simulink model "Controller_ABS_VLC_AYC_ALGO2"  (Simulink 8.7)
settings: Solver=ode3  SolverMode=SingleTasking  StartTime=0.0  StopTime=6  FixedStep=0.001  RelTol=1e-3
undefined symbols (not defined in the file): Beta_Err_P_Gain, Cf, Cr, f_R_SA_cutoff, f_R_SA_cutoff_HP, f_WT_cutoff, f_YAW_cutoff, Fz, g, Kc1, Kc2, KX0, KX1, KX2, Lf, Lr, Lw, R_SA_Alpha_Gain, R_SA_Beta_Gain, R_SA_D_Gain, R_SA_P_Gain, SE_Alpha_Gain, SE_Beta_Gain, SE_D_Gain, SE_P_Gain, SR_Lim_n, SR_Lim_p, STA_BETA, STA_BETA_a, STA_DBETA, STA_DBETA_a, STA_DYE, STA_DYE_a, STA_OUT_K, STA_OUT_K_a, STA_OUT_K_BETA, STA_YE, STA_YE_a, T_Avail, Target_SR, Tau_Yaw, V_SA_D_Gain, V_SA_P_Gain, WT_P_Gain, YAW_Alpha_Gain, YAW_Beta_Gain, Yaw_Ctrl_Gain_SMCC, YAW_D_Gain, Yaw_Err_P_Gain, YAW_Int_Gain, YAW_P_Gain, YAW_Prop_Gain
libraries: dspindex x4
settings Model: MinMaxOverflowLogging=ForceOff  Creator=MR Spyder  LastModifiedBy=MR Spyder
settings DataIOCC: SignalLoggingSaveFormat=ModelDataLogs  SaveOutput=off  SaveTime=off
settings OptimizationCC: DefaultParameterBehavior=Inlined  ExpressionDepthLimit=2147483647
settings DebuggingCC: SolverPrmCheckMsg=warning  FcnCallInpInsideContextMsg=EnableAllAsWarning  StateNameClashWarn=warning
settings GRTTargetCC: CombineOutputUpdateFcns=off  GRTInterface=on

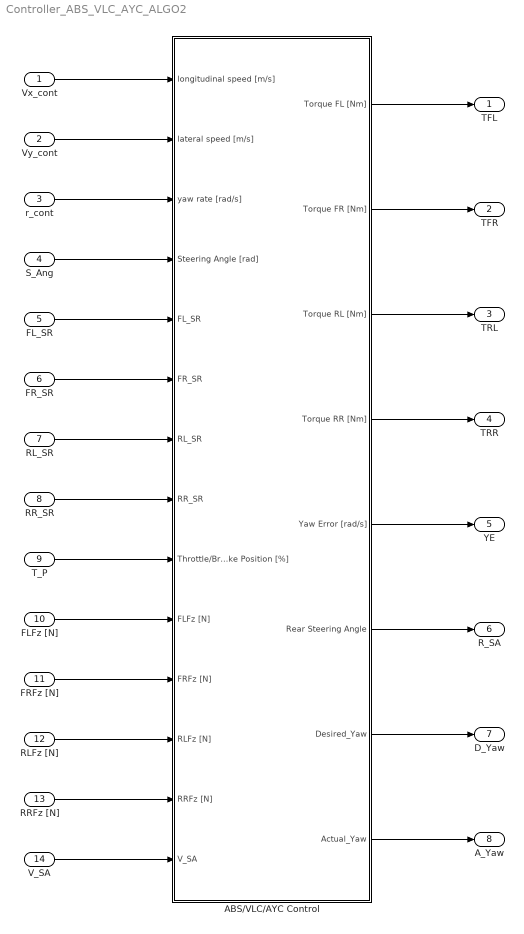
== system Controller_ABS_VLC_AYC_ALGO2 ==
  Vx_cont : Inport
  Vy_cont : Inport  Port=2
  r_cont : Inport  Port=3
  S_Ang : Inport  Port=4
  FL_SR : Inport  Port=5
  FR_SR : Inport  Port=6
  RL_SR : Inport  Port=7
  RR_SR : Inport  Port=8
  T_P : Inport  Port=9
  FLFz [N] : Inport  Port=10
  FRFz [N] : Inport  Port=11
  RLFz [N] : Inport  Port=12
  RRFz [N] : Inport  Port=13
  V_SA : Inport  Port=14
  ABS/VLC/AYC Control : Subsystem
  TFL : Outport
  TFR : Outport  Port=2
  TRL : Outport  Port=3
  TRR : Outport  Port=4
  YE : Outport  Port=5
  R_SA : Outport  Port=6
  D_Yaw : Outport  Port=7
  A_Yaw : Outport  Port=8
  wires:
  T_P/1 -> ABS/VLC/AYC Control/9(Throttle/Brake Position [%])
  ABS/VLC/AYC Control/1(Torque FL [Nm]) -> TFL/1
  ABS/VLC/AYC Control/2(Torque FR [Nm]) -> TFR/1
  ABS/VLC/AYC Control/3(Torque RL [Nm]) -> TRL/1
  ABS/VLC/AYC Control/4(Torque RR [Nm]) -> TRR/1
  FL_SR/1 -> ABS/VLC/AYC Control/5(FL_SR)
  FR_SR/1 -> ABS/VLC/AYC Control/6(FR_SR)
  RL_SR/1 -> ABS/VLC/AYC Control/7(RL_SR)
  RR_SR/1 -> ABS/VLC/AYC Control/8(RR_SR)
  r_cont/1 -> ABS/VLC/AYC Control/3(yaw rate [rad/s])
  Vy_cont/1 -> ABS/VLC/AYC Control/2(lateral speed [m/s])
  Vx_cont/1 -> ABS/VLC/AYC Control/1(longitudinal speed [m/s])
  S_Ang/1 -> ABS/VLC/AYC Control/4(Steering Angle [rad])
  ABS/VLC/AYC Control/5(Yaw Error [rad/s]) -> YE/1
  FLFz [N]/1 -> ABS/VLC/AYC Control/10(FLFz [N])
  FRFz [N]/1 -> ABS/VLC/AYC Control/11(FRFz [N])
  RLFz [N]/1 -> ABS/VLC/AYC Control/12(RLFz [N])
  RRFz [N]/1 -> ABS/VLC/AYC Control/13(RRFz [N])
  ABS/VLC/AYC Control/6(Rear Steering Angle) -> R_SA/1
  V_SA/1 -> ABS/VLC/AYC Control/14(V_SA)
  ABS/VLC/AYC Control/7(Desired_Yaw) -> D_Yaw/1
  ABS/VLC/AYC Control/8(Actual_Yaw) -> A_Yaw/1

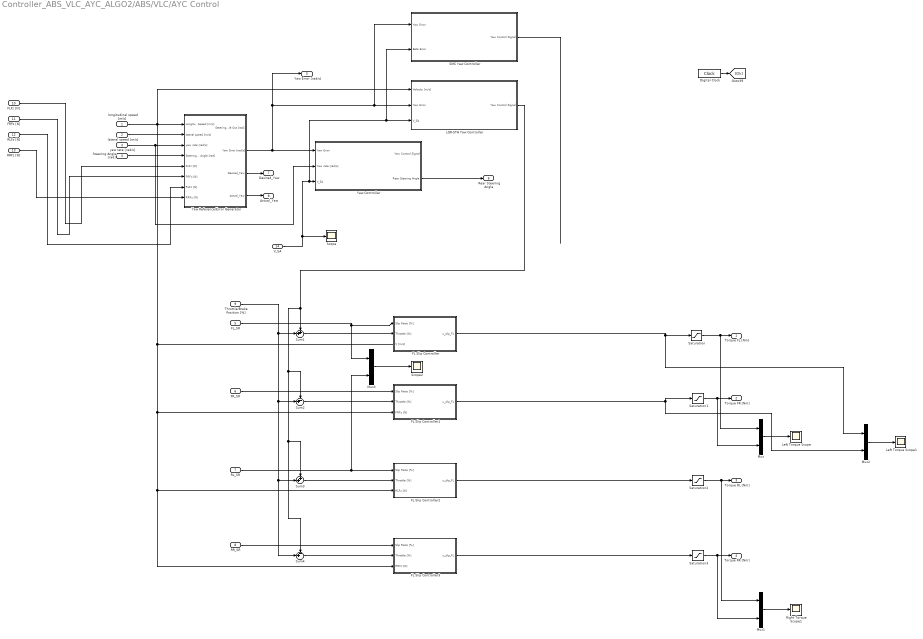
== system Controller_ABS_VLC_AYC_ALGO2/ABS/VLC/AYC Control ==
  longitudinal speed [m/s] : Inport
  lateral speed [m/s] : Inport  Port=2
  yaw rate [rad/s] : Inport  Port=3
  Steering Angle [rad] : Inport  Port=4
  FL_SR : Inport  Port=5
  FR_SR : Inport  Port=6
  RL_SR : Inport  Port=7
  RR_SR : Inport  Port=8
  Throttle/Brake Position [%] : Inport  Port=9
  FLFz [N] : Inport  Port=10
  FRFz [N] : Inport  Port=11
  RLFz [N] : Inport  Port=12
  RRFz [N] : Inport  Port=13
  V_SA : Inport  Port=14
  Digital Clock : DigitalClock  SampleTime=0.001
  FL Slip Controller : Subsystem
  FL Slip Controller1 : Subsystem
  FL Slip Controller2 : Subsystem
  FL Slip Controller3 : Subsystem
  LQR-STA Yaw Controller : Subsystem
  Left Torque Scope : Scope
  Left Torque Scope1 : Scope
  Mux{,1..3} (4 alike) : Mux  Inputs=2
  Right Torque Scope1 : Scope
  SMC Yaw Controller : Subsystem
  Saturation{,1..3} (4 alike) : Saturate  UpperLimit=T_Avail  LowerLimit=-T_Avail  LinearizeAsGain=off
  Scope : Scope
  Scope2 : Scope
  Sum1 : Sum  Inputs=++|
  Sum2 : Sum  Inputs=-+|
  Sum3 : Sum  Inputs=++|
  Sum4 : Sum  Inputs=-+|
  Yaw Controller : Subsystem
  Yaw Reference/Error Generator : Subsystem
  Torque FL [Nm] : Outport
  Torque FR [Nm] : Outport  Port=2
  Torque RL [Nm] : Outport  Port=3
  Torque RR [Nm] : Outport  Port=4
  Yaw Error [rad/s] : Outport  Port=5
  Rear Steering Angle : Outport  Port=6
  Desired_Yaw : Outport  Port=7
  Actual_Yaw : Outport  Port=8
  wires:
  Mux/1 -> Left Torque Scope/1
  Throttle/Brake Position [%]/1 -> Sum1/2, Sum2/2, Sum4/2, Sum3/2
  Mux1/1 -> Right Torque Scope1/1
  FL_SR/1 -> FL Slip Controller/1(Slip Ratio [%]), Mux3/1
  RL_SR/1 -> Mux3/2, FL Slip Controller2/1(Slip Ratio [%])
  RR_SR/1 -> FL Slip Controller3/1(Slip Ratio [%])
  Digital Clock/1 -> [Clk]
  FL Slip Controller/1(u_slip_FL) -> Mux2/1, Saturation/1
  FL Slip Controller1/1(u_slip_FL) -> Saturation1/1, Mux2/2
  FL Slip Controller2/1(u_slip_FL) -> Saturation2/1
  FL Slip Controller3/1(u_slip_FL) -> Saturation3/1
  LQR-STA Yaw Controller/1(Yaw Control Signal) -> Sum2/1, Sum3/1, Sum4/1, Sum1/1
  Saturation/1 -> Torque FL [Nm]/1, Mux/1
  Saturation1/1 -> Torque FR [Nm]/1, Mux/2
  Saturation2/1 -> Torque RL [Nm]/1, Mux1/1
  Saturation3/1 -> Torque RR [Nm]/1, Mux1/2
  Mux2/1 -> Left Torque Scope1/1
  Mux3/1 -> Scope2/1
  FR_SR/1 -> FL Slip Controller1/1(Slip Ratio [%])
  Sum1/1 -> FL Slip Controller/2(Throttle [%])
  Sum2/1 -> FL Slip Controller1/2(Throttle [%])
  Sum3/1 -> FL Slip Controller2/2(Throttle [%])
  Sum4/1 -> FL Slip Controller3/2(Throttle [%])
  yaw rate [rad/s]/1 -> Yaw Controller/2(Yaw rate [rad/s]), Yaw Reference/Error Generator/3(yaw rate [rad/s])
  Yaw Controller/2(Rear Steering Angle) -> Rear Steering Angle/1
  V_SA/1 -> Scope/1, SMC Yaw Controller/2(Beta Error), LQR-STA Yaw Controller/3(V_SA), Yaw Controller/3(V_SA)
  Yaw Reference/Error Generator/2(Yaw Error [rad/s]) -> Yaw Error [rad/s]/1, SMC Yaw Controller/1(Yaw Error), LQR-STA Yaw Controller/2(Yaw Error), Yaw Controller/1(Yaw Error)
  Yaw Reference/Error Generator/3(Desired_Yaw) -> Desired_Yaw/1
  Yaw Reference/Error Generator/4(Actual_Yaw) -> Actual_Yaw/1
  longitudinal speed [m/s]/1 -> FL Slip Controller1/3(FRFz [N]), FL Slip Controller3/3(RRFz [N]), FL Slip Controller2/3(RLFz [N]), LQR-STA Yaw Controller/1(Velocity [m/s]), Yaw Reference/Error Generator/1(Longitudinal Speed [m/s])
  lateral speed [m/s]/1 -> Yaw Reference/Error Generator/2(lateral speed [m/s])
  Steering Angle [rad]/1 -> Yaw Reference/Error Generator/4(Steering Angle [rad])
  FLFz [N]/1 -> Yaw Reference/Error Generator/5(FLFz [N])
  FRFz [N]/1 -> Yaw Reference/Error Generator/6(FRFz [N])
  RLFz [N]/1 -> Yaw Reference/Error Generator/7(RLFz [N])
  RRFz [N]/1 -> Yaw Reference/Error Generator/8(RRFz [N])
  SMC Yaw Controller/1(Yaw Control Signal) -> ?

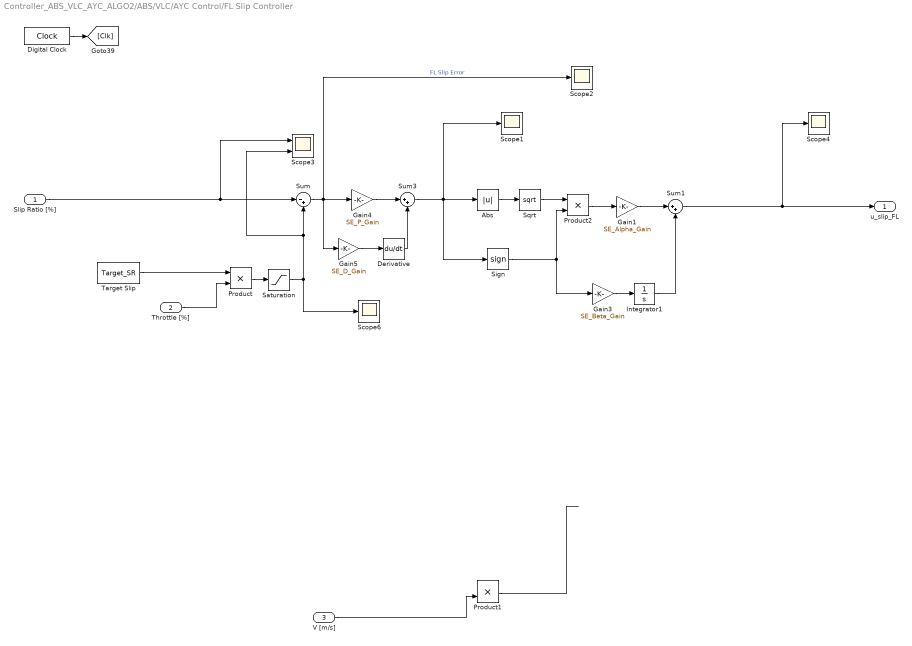
== system Controller_ABS_VLC_AYC_ALGO2/ABS/VLC/AYC Control/FL Slip Controller ==
  Slip Ratio [%] : Inport
  Throttle [%] : Inport  Port=2
  V [m/s] : Inport  Port=3
  Abs : Abs
  Derivative : Derivative
  Digital Clock : DigitalClock  SampleTime=0.001
  Gain1 : Gain  Gain=SE_Alpha_Gain
  Gain3 : Gain  Gain=SE_Beta_Gain
  Gain4 : Gain  Gain=SE_P_Gain
  Gain5 : Gain  Gain=SE_D_Gain
  Integrator1 : Integrator
  Product : Product
  Product1 : Product
  Product2 : Product
  Saturation : Saturate  UpperLimit=SR_Lim_p  LowerLimit=SR_Lim_n  LinearizeAsGain=off
  Scope{1..2,4,6} (4 alike) : Scope
  Scope3 : Scope  NumInputPorts=2
  Sign : Signum
  Sqrt : Sqrt  SaturateOnIntegerOverflow=on
  Sum : Sum  Inputs=|-+
  Sum1 : Sum  Inputs=|++
  Sum3 : Sum  Inputs=|++
  Target Slip : Constant  Value=Target_SR
  u_slip_FL : Outport
  wires:
  Digital Clock/1 -> [Clk]
  Sqrt/1 -> Product2/1
  Sum1/1 -> Scope4/1, u_slip_FL/1
  Slip Ratio [%]/1 -> Sum/1, Scope3/1
  Throttle [%]/1 -> Product/2
  Product/1 -> Saturation/1
  Target Slip/1 -> Product/1
  Sum/1 -> Gain5/1, Gain4/1, Scope2/1  "FL Slip Error"
  Product2/1 -> Gain1/1
  Abs/1 -> Sqrt/1
  Sign/1 -> Gain3/1, Product2/2
  Sum3/1 -> Scope1/1, Sign/1, Abs/1
  Integrator1/1 -> Sum1/2
  Gain1/1 -> Sum1/1
  Gain3/1 -> Integrator1/1
  Gain4/1 -> Sum3/1
  Derivative/1 -> Sum3/2
  Gain5/1 -> Derivative/1
  Saturation/1 -> Scope6/1, Scope3/2, Sum/2
  ? -> Product1/1
  V [m/s]/1 -> Product1/2
  Product1/1 -> ?

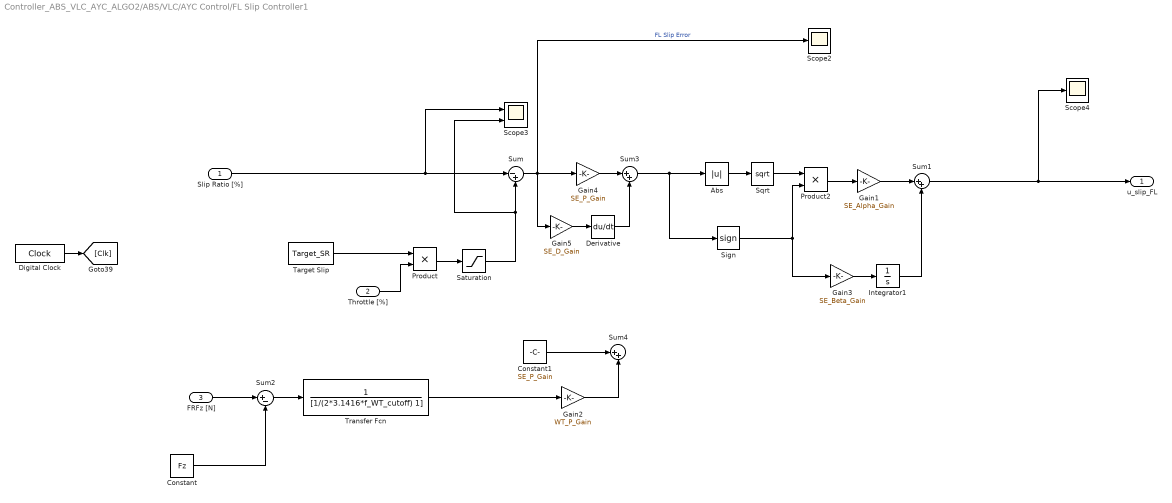
== system Controller_ABS_VLC_AYC_ALGO2/ABS/VLC/AYC Control/FL Slip Controller1 ==
  Slip Ratio [%] : Inport
  Throttle [%] : Inport  Port=2
  FRFz [N] : Inport  Port=3
  Abs : Abs
  Constant : Constant  Value=Fz
  Constant1 : Constant  Value=SE_P_Gain
  Derivative : Derivative
  Digital Clock : DigitalClock  SampleTime=0.001
  Gain1 : Gain  Gain=SE_Alpha_Gain
  Gain2 : Gain  Gain=WT_P_Gain
  Gain3 : Gain  Gain=SE_Beta_Gain
  Gain4 : Gain  Gain=SE_P_Gain
  Gain5 : Gain  Gain=SE_D_Gain
  Integrator1 : Integrator
  Product : Product
  Product2 : Product
  Saturation : Saturate  UpperLimit=SR_Lim_p  LowerLimit=SR_Lim_n  LinearizeAsGain=off
  Scope2 : Scope
  Scope3 : Scope  NumInputPorts=2
  Scope4 : Scope
  Sign : Signum
  Sqrt : Sqrt  SaturateOnIntegerOverflow=on
  Sum : Sum  Inputs=|-+
  Sum1 : Sum  Inputs=|++
  Sum2 : Sum  Inputs=|+-
  Sum3 : Sum  Inputs=|++
  Sum4 : Sum  Inputs=|++
  Target Slip : Constant  Value=Target_SR
  Transfer Fcn : TransferFcn  Denominator=[1/(2*3.1416*f_WT_cutoff) 1]
  u_slip_FL : Outport
  wires:
  Sqrt/1 -> Product2/1
  Digital Clock/1 -> [Clk]
  Sum1/1 -> Scope4/1, u_slip_FL/1
  Slip Ratio [%]/1 -> Sum/1, Scope3/1
  Throttle [%]/1 -> Product/2
  Product/1 -> Saturation/1
  Target Slip/1 -> Product/1
  FRFz [N]/1 -> Sum2/1
  Transfer Fcn/1 -> Gain2/1
  Constant/1 -> Sum2/2
  Sum2/1 -> Transfer Fcn/1
  Sum/1 -> Gain5/1, Gain4/1, Scope2/1  "FL Slip Error"
  Gain2/1 -> Sum4/2
  Constant1/1 -> Sum4/1
  Product2/1 -> Gain1/1
  Abs/1 -> Sqrt/1
  Sign/1 -> Product2/2, Gain3/1
  Derivative/1 -> Sum3/2
  Sum3/1 -> Sign/1, Abs/1
  Integrator1/1 -> Sum1/2
  Gain1/1 -> Sum1/1
  Gain3/1 -> Integrator1/1
  Gain4/1 -> Sum3/1
  Gain5/1 -> Derivative/1
  Saturation/1 -> Scope3/2, Sum/2

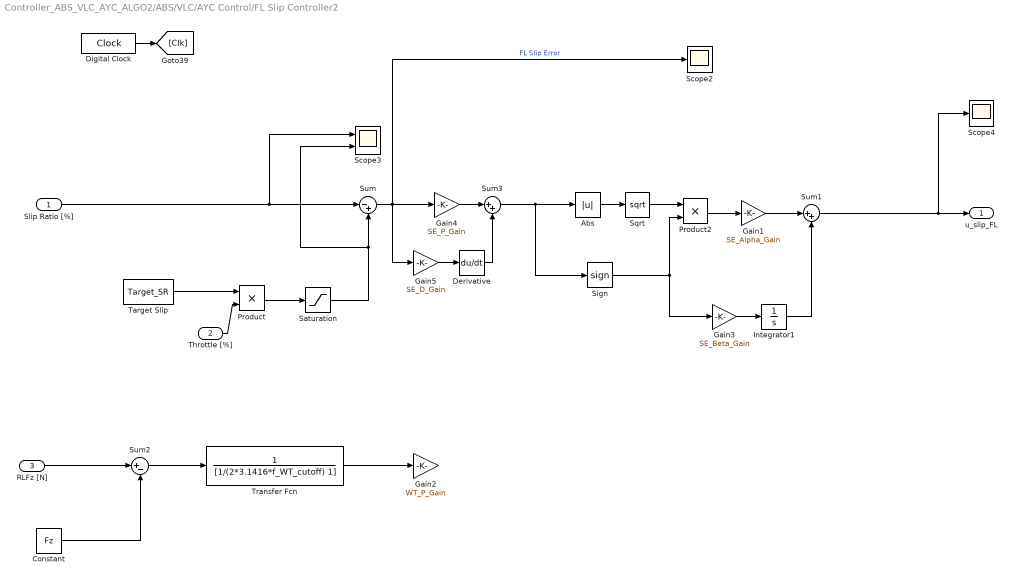
== system Controller_ABS_VLC_AYC_ALGO2/ABS/VLC/AYC Control/FL Slip Controller2 ==
  Slip Ratio [%] : Inport
  Throttle [%] : Inport  Port=2
  RLFz [N] : Inport  Port=3
  Abs : Abs
  Constant : Constant  Value=Fz
  Derivative : Derivative
  Digital Clock : DigitalClock  SampleTime=0.001
  Gain1 : Gain  Gain=SE_Alpha_Gain
  Gain2 : Gain  Gain=WT_P_Gain
  Gain3 : Gain  Gain=SE_Beta_Gain
  Gain4 : Gain  Gain=SE_P_Gain
  Gain5 : Gain  Gain=SE_D_Gain
  Integrator1 : Integrator
  Product : Product
  Product2 : Product
  Saturation : Saturate  UpperLimit=SR_Lim_p  LowerLimit=SR_Lim_n  LinearizeAsGain=off
  Scope2 : Scope
  Scope3 : Scope  NumInputPorts=2
  Scope4 : Scope
  Sign : Signum
  Sqrt : Sqrt  SaturateOnIntegerOverflow=on
  Sum : Sum  Inputs=|-+
  Sum1 : Sum  Inputs=|++
  Sum2 : Sum  Inputs=|+-
  Sum3 : Sum  Inputs=|++
  Target Slip : Constant  Value=Target_SR
  Transfer Fcn : TransferFcn  Denominator=[1/(2*3.1416*f_WT_cutoff) 1]
  u_slip_FL : Outport
  wires:
  Digital Clock/1 -> [Clk]
  RLFz [N]/1 -> Sum2/1
  Transfer Fcn/1 -> Gain2/1
  Constant/1 -> Sum2/2
  Sum2/1 -> Transfer Fcn/1
  Sqrt/1 -> Product2/1
  Sum1/1 -> u_slip_FL/1, Scope4/1
  Slip Ratio [%]/1 -> Sum/1, Scope3/1
  Throttle [%]/1 -> Product/2
  Product/1 -> Saturation/1
  Target Slip/1 -> Product/1
  Sum/1 -> Gain5/1, Gain4/1, Scope2/1  "FL Slip Error"
  Product2/1 -> Gain1/1
  Abs/1 -> Sqrt/1
  Sign/1 -> Product2/2, Gain3/1
  Derivative/1 -> Sum3/2
  Sum3/1 -> Sign/1, Abs/1
  Integrator1/1 -> Sum1/2
  Gain1/1 -> Sum1/1
  Gain3/1 -> Integrator1/1
  Gain4/1 -> Sum3/1
  Gain5/1 -> Derivative/1
  Saturation/1 -> Scope3/2, Sum/2

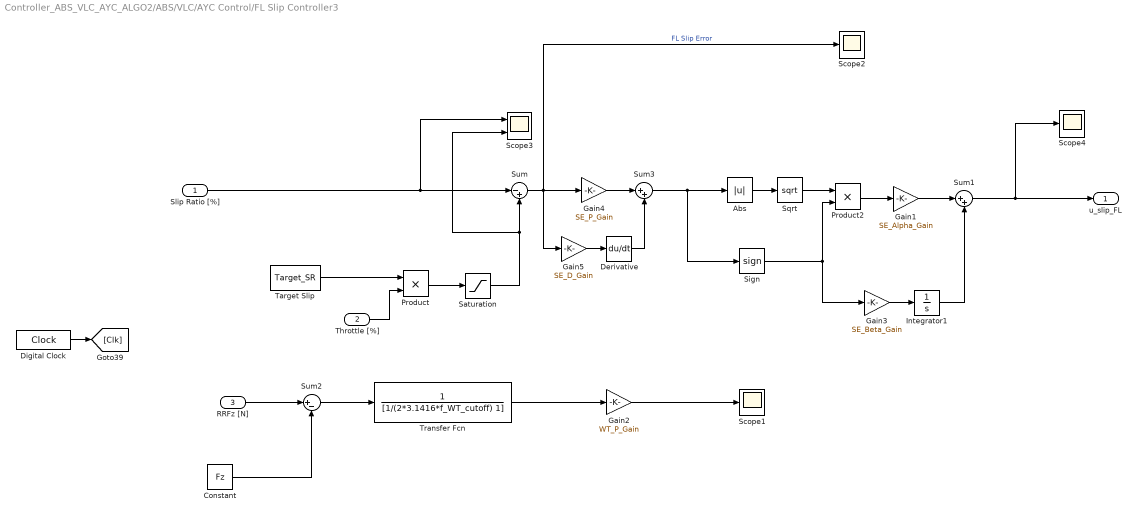
== system Controller_ABS_VLC_AYC_ALGO2/ABS/VLC/AYC Control/FL Slip Controller3 ==
  Slip Ratio [%] : Inport
  Throttle [%] : Inport  Port=2
  RRFz [N] : Inport  Port=3
  Abs : Abs
  Constant : Constant  Value=Fz
  Derivative : Derivative
  Digital Clock : DigitalClock  SampleTime=0.001
  Gain1 : Gain  Gain=SE_Alpha_Gain
  Gain2 : Gain  Gain=WT_P_Gain
  Gain3 : Gain  Gain=SE_Beta_Gain
  Gain4 : Gain  Gain=SE_P_Gain
  Gain5 : Gain  Gain=SE_D_Gain
  Integrator1 : Integrator
  Product : Product
  Product2 : Product
  Saturation : Saturate  UpperLimit=SR_Lim_p  LowerLimit=SR_Lim_n  LinearizeAsGain=off
  Scope1 : Scope
  Scope2 : Scope
  Scope3 : Scope  NumInputPorts=2
  Scope4 : Scope
  Sign : Signum
  Sqrt : Sqrt  SaturateOnIntegerOverflow=on
  Sum : Sum  Inputs=|-+
  Sum1 : Sum  Inputs=|++
  Sum2 : Sum  Inputs=|+-
  Sum3 : Sum  Inputs=|++
  Target Slip : Constant  Value=Target_SR
  Transfer Fcn : TransferFcn  Denominator=[1/(2*3.1416*f_WT_cutoff) 1]
  u_slip_FL : Outport
  wires:
  Digital Clock/1 -> [Clk]
  RRFz [N]/1 -> Sum2/1
  Transfer Fcn/1 -> Gain2/1
  Constant/1 -> Sum2/2
  Sum2/1 -> Transfer Fcn/1
  Sqrt/1 -> Product2/1
  Sum1/1 -> u_slip_FL/1, Scope4/1
  Slip Ratio [%]/1 -> Sum/1, Scope3/1
  Throttle [%]/1 -> Product/2
  Product/1 -> Saturation/1
  Target Slip/1 -> Product/1
  Sum/1 -> Gain5/1, Gain4/1, Scope2/1  "FL Slip Error"
  Product2/1 -> Gain1/1
  Abs/1 -> Sqrt/1
  Sign/1 -> Product2/2, Gain3/1
  Derivative/1 -> Sum3/2
  Sum3/1 -> Sign/1, Abs/1
  Integrator1/1 -> Sum1/2
  Gain1/1 -> Sum1/1
  Gain3/1 -> Integrator1/1
  Gain2/1 -> Scope1/1
  Gain4/1 -> Sum3/1
  Gain5/1 -> Derivative/1
  Saturation/1 -> Scope3/2, Sum/2

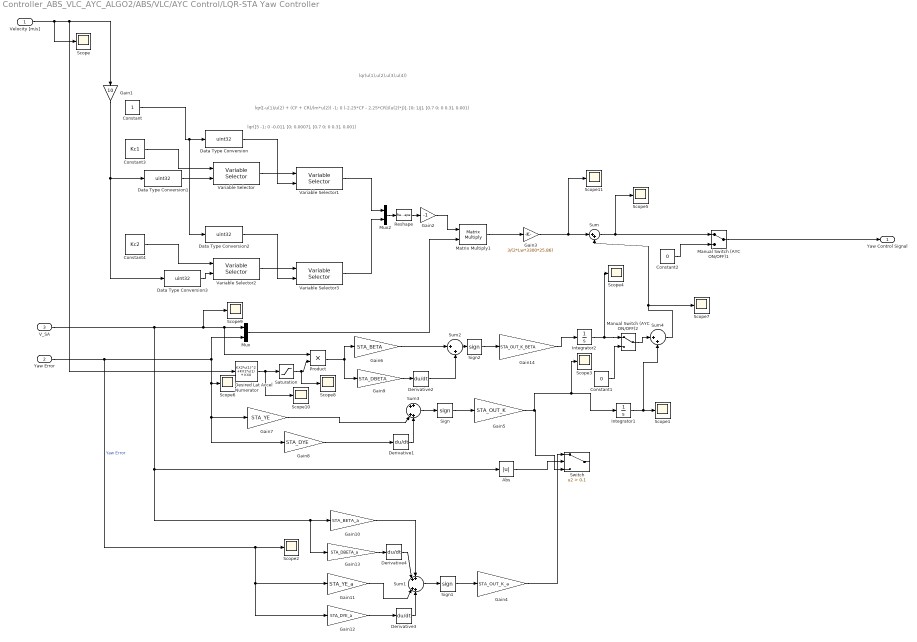
== system Controller_ABS_VLC_AYC_ALGO2/ABS/VLC/AYC Control/LQR-STA Yaw Controller ==
  note: lqr([5 -1; 0 -0.01], [0; 0.0007], [0.7 0; 0 0.3], 0.001)
  note: lqr([-u(1)/u(2) + (CF + CR)/(m*u(2)) -1; 0 (-2.25*CF - 2.25*CR)/(u(2)*J)], [0; 1/J], [0.7 0; 0 0.3], 0.001)
  note: lqr(u(1),u(2),u(3),u(4))
  Velocity [m/s] : Inport
  Yaw Error : Inport  Port=2
  V_SA : Inport  Port=3
  Abs : Abs
  Constant : Constant
  Constant1 : Constant  Value=0
  Constant2 : Constant  Value=0
  Constant3 : Constant  Value=Kc1
  Constant4 : Constant  Value=Kc2
  Data Type Conversion{,1..3} (4 alike) : DataTypeConversion  OutDataTypeStr=uint32
  Derivative{1..4} (4 alike) : Derivative
  Desired Lat Accel Numerator : Fcn  Expr=KX2*u(1)^2 +KX1*u(1) + KX0
  Gain1 : Gain  Gain=10
  Gain10 : Gain  Gain=STA_BETA_a
  Gain11 : Gain  Gain=STA_YE_a
  Gain12 : Gain  Gain=STA_DYE_a
  Gain13 : Gain  Gain=STA_DBETA_a
  Gain14 : Gain  Gain=STA_OUT_K_BETA
  Gain2 : Gain  Gain=-1
  Gain3 : Gain  Gain=3/(2*Lw*3300*25.86)
  Gain4 : Gain  Gain=STA_OUT_K_a
  Gain5 : Gain  Gain=STA_OUT_K
  Gain6 : Gain  Gain=STA_BETA
  Gain7 : Gain  Gain=STA_YE
  Gain8 : Gain  Gain=STA_DYE
  Gain9 : Gain  Gain=STA_DBETA
  Integrator1 : Integrator
  Integrator2 : Integrator
  Manual Switch (AYC ON/OFF)1 : ManualSwitch
  Manual Switch (AYC ON/OFF)2 : ManualSwitch
  Matrix Multiply1 : Product  Multiplication=Matrix(*)
  Mux : Mux  Inputs=2
  Mux2 : Mux  Inputs=2
  Product : Product
  Reshape : Reshape  OutputDimensionality=Row vector (2-D)
  Saturation : Saturate  UpperLimit=1  LowerLimit=0
  Scope{,1..11} (12 alike) : Scope
  Sign : Signum
  Sign1 : Signum
  Sign2 : Signum
  Sum : Sum  Inputs=|++
  Sum1 : Sum  Inputs=++||++
  Sum2 : Sum  Inputs=|++
  Sum3 : Sum  Inputs=++||++
  Sum4 : Sum  Inputs=|++
  Switch : Switch  Criteria=u2 > Threshold  Threshold=0.1
  Variable Selector : dspindex/Variable Selector  NumInputs=1  rowsOrCols=Rows  IdxMode=Variable  Elements=[1 3]  ZerOneIdxMode=One-based  errmode=Clip Index  FillMode=on  FillValues=0
  Variable Selector1 : dspindex/Variable Selector  NumInputs=1  rowsOrCols=Columns  IdxMode=Variable  Elements=[1 3]  ZerOneIdxMode=One-based  errmode=Clip Index  FillMode=on  FillValues=0
  Variable Selector2 : dspindex/Variable Selector  NumInputs=1  rowsOrCols=Rows  IdxMode=Variable  Elements=[1 3]  ZerOneIdxMode=One-based  errmode=Clip Index  FillMode=on  FillValues=0
  Variable Selector3 : dspindex/Variable Selector  NumInputs=1  rowsOrCols=Columns  IdxMode=Variable  Elements=[1 3]  ZerOneIdxMode=One-based  errmode=Clip Index  FillMode=on  FillValues=0
  Yaw Control Signal : Outport
  wires:
  Velocity [m/s]/1 -> Scope/1, Desired Lat Accel Numerator/1, Gain1/1
  Constant3/1 -> Variable Selector/1
  Variable Selector/1 -> Variable Selector1/1
  Variable Selector1/1 -> Mux2/1
  Data Type Conversion/1 -> Variable Selector1/2
  Data Type Conversion1/1 -> Variable Selector/2
  Constant4/1 -> Variable Selector2/1
  Variable Selector2/1 -> Variable Selector3/1
  Data Type Conversion2/1 -> Variable Selector3/2
  Data Type Conversion3/1 -> Variable Selector2/2
  Constant/1 -> Data Type Conversion2/1, Data Type Conversion/1
  Gain1/1 -> Data Type Conversion1/1, Data Type Conversion3/1
  Variable Selector3/1 -> Mux2/2
  Matrix Multiply1/1 -> Gain3/1
  Mux2/1 -> Reshape/1
  Gain2/1 -> Matrix Multiply1/1
  Reshape/1 -> Gain2/1
  Mux/1 -> Matrix Multiply1/2
  Sum/1 -> Manual Switch (AYC ON/OFF)1/1, Scope5/1
  Gain3/1 -> Scope11/1, Sum/1
  Sign/1 -> Gain5/1
  Gain7/1 -> Sum3/3
  Derivative1/1 -> Sum3/4
  Gain8/1 -> Derivative1/1
  Sum3/1 -> Sign/1
  Gain9/1 -> Derivative2/1
  Constant2/1 -> Manual Switch (AYC ON/OFF)1/2
  Manual Switch (AYC ON/OFF)1/1 -> Yaw Control Signal/1
  Integrator1/1 -> Scope1/1, Sum4/2
  Gain5/1 -> Scope3/1, Integrator1/1, Switch/3
  Yaw Error/1 -> Scope2/1, Gain11/1, Gain12/1, Scope6/1, Gain7/1, Gain8/1, Mux/2  "Yaw Error"
  Sign1/1 -> Gain4/1
  Gain11/1 -> Sum1/3
  Derivative3/1 -> Sum1/4
  Gain12/1 -> Derivative3/1
  Sum1/1 -> Sign1/1
  Gain13/1 -> Derivative4/1
  Gain10/1 -> Sum1/1
  Derivative4/1 -> Sum1/2
  V_SA/1 -> Abs/1, Gain13/1, Gain10/1, Scope9/1, Product/1, Mux/1
  Gain4/1 -> Switch/1
  Abs/1 -> Switch/2
  Integrator2/1 -> Manual Switch (AYC ON/OFF)2/1, Scope4/1
  Sum4/1 -> Scope7/1, Sum/2
  Manual Switch (AYC ON/OFF)2/1 -> Sum4/1
  Constant1/1 -> Manual Switch (AYC ON/OFF)2/2
  Product/1 -> Gain9/1, Gain6/1
  Desired Lat Accel Numerator/1 -> Scope10/1, Saturation/1
  Saturation/1 -> Scope8/1, Product/2
  Derivative2/1 -> Sum2/2
  Gain6/1 -> Sum2/1
  Sum2/1 -> Sign2/1
  Sign2/1 -> Gain14/1
  Gain14/1 -> Integrator2/1

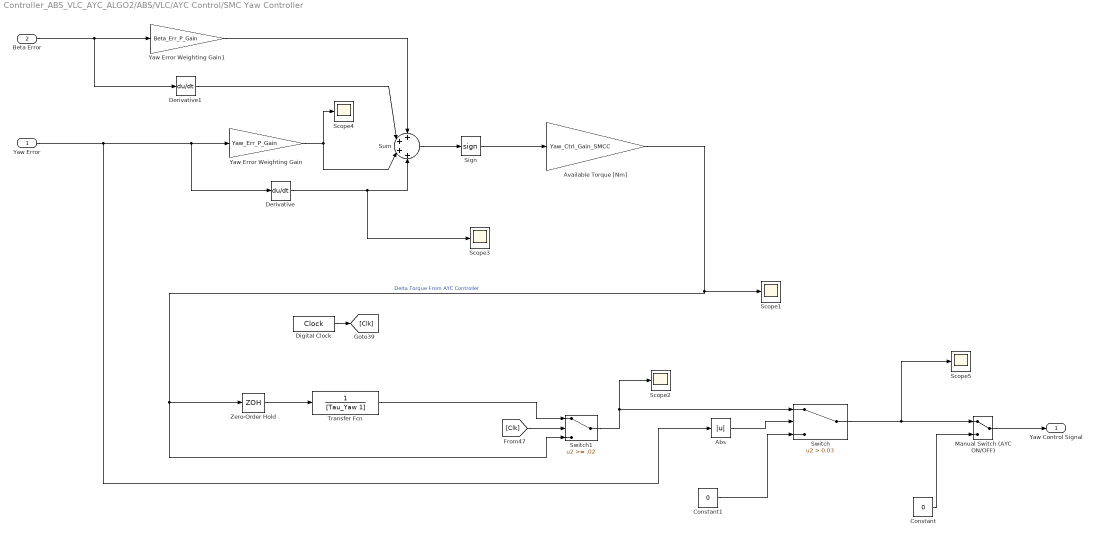
== system Controller_ABS_VLC_AYC_ALGO2/ABS/VLC/AYC Control/SMC Yaw Controller ==
  Yaw Error : Inport
  Beta Error : Inport  Port=2
  Abs : Abs
  Available Torque [Nm] : Gain  Gain=Yaw_Ctrl_Gain_SMCC
  Constant : Constant  Value=0
  Constant1 : Constant  Value=0
  Derivative : Derivative
  Derivative1 : Derivative
  Digital Clock : DigitalClock  SampleTime=0.001
  Manual Switch (AYC ON/OFF) : ManualSwitch
  Scope{1..5} (5 alike) : Scope
  Sign : Signum
  Sum : Sum  Inputs=+|+|+|+
  Switch : Switch  Criteria=u2 > Threshold  Threshold=0.03
  Switch1 : Switch  Threshold=.02
  Transfer Fcn : TransferFcn  Denominator=[Tau_Yaw 1]
  Yaw Error Weighting Gain : Gain  Gain=Yaw_Err_P_Gain
  Yaw Error Weighting Gain1 : Gain  Gain=Beta_Err_P_Gain
  Zero-Order Hold : ZeroOrderHold  SampleTime=.001
  Yaw Control Signal : Outport
  wires:
  Yaw Error Weighting Gain/1 -> Sum/3, Scope4/1
  Sign/1 -> Available Torque [Nm]/1
  Available Torque [Nm]/1 -> Zero-Order Hold/1, Switch1/3, Scope1/1  "Delta Torque From AYC Controller"
  [Clk] -> Switch1/2
  Transfer Fcn/1 -> Switch1/1
  Digital Clock/1 -> [Clk]
  Sum/1 -> Sign/1
  Constant/1 -> Manual Switch (AYC ON/OFF)/2
  Manual Switch (AYC ON/OFF)/1 -> Yaw Control Signal/1
  Yaw Error/1 -> Abs/1, Derivative/1, Yaw Error Weighting Gain/1
  Switch1/1 -> Switch/1, Scope2/1
  Zero-Order Hold/1 -> Transfer Fcn/1
  Switch/1 -> Scope5/1, Manual Switch (AYC ON/OFF)/1
  Constant1/1 -> Switch/3
  Abs/1 -> Switch/2
  Derivative/1 -> Sum/4, Scope3/1
  Beta Error/1 -> Derivative1/1, Yaw Error Weighting Gain1/1
  Yaw Error Weighting Gain1/1 -> Sum/1
  Derivative1/1 -> Sum/2

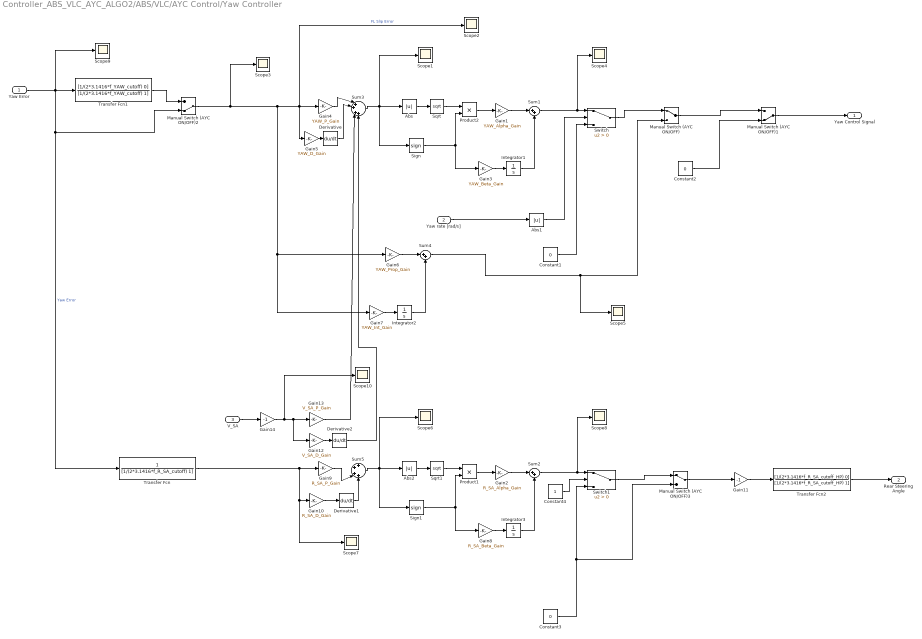
== system Controller_ABS_VLC_AYC_ALGO2/ABS/VLC/AYC Control/Yaw Controller ==
  Yaw Error : Inport
  Yaw rate [rad/s] : Inport  Port=2
  V_SA : Inport  Port=3
  Abs : Abs
  Abs1 : Abs
  Abs2 : Abs
  Constant1 : Constant  Value=0
  Constant2 : Constant  Value=0
  Constant3 : Constant  Value=0
  Constant4 : Constant
  Derivative : Derivative
  Derivative1 : Derivative
  Derivative2 : Derivative
  Gain1 : Gain  Gain=YAW_Alpha_Gain
  Gain10 : Gain  Gain=R_SA_D_Gain
  Gain11 : Gain  Gain=-1
  Gain12 : Gain  Gain=V_SA_D_Gain
  Gain13 : Gain  Gain=V_SA_P_Gain
  Gain14 : Gain  Gain=-1
  Gain2 : Gain  Gain=R_SA_Alpha_Gain
  Gain3 : Gain  Gain=YAW_Beta_Gain
  Gain4 : Gain  Gain=YAW_P_Gain
  Gain5 : Gain  Gain=YAW_D_Gain
  Gain6 : Gain  Gain=YAW_Prop_Gain
  Gain7 : Gain  Gain=YAW_Int_Gain
  Gain8 : Gain  Gain=R_SA_Beta_Gain
  Gain9 : Gain  Gain=R_SA_P_Gain
  Integrator1 : Integrator
  Integrator2 : Integrator
  Integrator3 : Integrator
  Manual Switch (AYC ON/OFF) : ManualSwitch
  Manual Switch (AYC ON/OFF)1 : ManualSwitch  CurrentSetting=0
  Manual Switch (AYC ON/OFF)2 : ManualSwitch  CurrentSetting=0
  Manual Switch (AYC ON/OFF)3 : ManualSwitch
  Product1 : Product
  Product2 : Product
  Scope{1..10} (10 alike) : Scope
  Sign : Signum
  Sign1 : Signum
  Sqrt : Sqrt  SaturateOnIntegerOverflow=on
  Sqrt1 : Sqrt  SaturateOnIntegerOverflow=on
  Sum1 : Sum  Inputs=|++
  Sum2 : Sum  Inputs=|++
  Sum3 : Sum  Inputs=|++|++
  Sum4 : Sum  Inputs=|++
  Sum5 : Sum  Inputs=++|++
  Switch : Switch  Criteria=u2 > Threshold
  Switch1 : Switch  Criteria=u2 > Threshold
  Transfer Fcn : TransferFcn  Denominator=[1/(2*3.1416*f_R_SA_cutoff) 1]
  Transfer Fcn1 : TransferFcn  Numerator=[1/(2*3.1416*f_YAW_cutoff) 0]  Denominator=[1/(2*3.1416*f_YAW_cutoff) 1]
  Transfer Fcn2 : TransferFcn  Numerator=[1/(2*3.1416*f_R_SA_cutoff_HP) 0]  Denominator=[1/(2*3.1416*f_R_SA_cutoff_HP) 1]
  Yaw Control Signal : Outport
  Rear Steering Angle : Outport  Port=2
  wires:
  Sum4/1 -> Scope5/1, Manual Switch (AYC ON/OFF)/2
  Manual Switch (AYC ON/OFF)/1 -> Manual Switch (AYC ON/OFF)1/1
  Sqrt/1 -> Product2/1
  Sum1/1 -> Scope4/1, Switch/1
  Product2/1 -> Gain1/1
  Abs/1 -> Sqrt/1
  Sign/1 -> Product2/2, Gain3/1
  Sum3/1 -> Scope1/1, Sign/1, Abs/1
  Integrator1/1 -> Sum1/2
  Gain1/1 -> Sum1/1
  Gain3/1 -> Integrator1/1
  Gain4/1 -> Sum3/1
  Derivative/1 -> Sum3/2
  Gain5/1 -> Derivative/1
  Switch/1 -> Manual Switch (AYC ON/OFF)/1
  Constant1/1 -> Switch/3
  Abs1/1 -> Switch/2
  Manual Switch (AYC ON/OFF)2/1 -> Scope3/1, Gain7/1, Gain6/1, Gain5/1, Gain4/1, Scope2/1  "FL Slip Error"
  Integrator2/1 -> Sum4/2
  Gain6/1 -> Sum4/1
  Gain7/1 -> Integrator2/1
  Constant2/1 -> Manual Switch (AYC ON/OFF)1/2
  Sqrt1/1 -> Product1/1
  Sum2/1 -> Scope8/1, Switch1/1
  Product1/1 -> Gain2/1
  Abs2/1 -> Sqrt1/1
  Sign1/1 -> Product1/2, Gain8/1
  Sum5/1 -> Scope6/1, Sign1/1, Abs2/1
  Integrator3/1 -> Sum2/2
  Gain2/1 -> Sum2/1
  Gain8/1 -> Integrator3/1
  Gain9/1 -> Sum5/3
  Derivative1/1 -> Sum5/4
  Gain10/1 -> Derivative1/1
  Yaw rate [rad/s]/1 -> Abs1/1
  Constant3/1 -> Manual Switch (AYC ON/OFF)3/2, Switch1/3
  Yaw Error/1 -> Scope9/1, Transfer Fcn/1, Manual Switch (AYC ON/OFF)2/2, Transfer Fcn1/1  "Yaw Error"
  Transfer Fcn1/1 -> Manual Switch (AYC ON/OFF)2/1
  Constant4/1 -> Switch1/2
  Switch1/1 -> Manual Switch (AYC ON/OFF)3/1
  Manual Switch (AYC ON/OFF)3/1 -> Gain11/1
  Gain11/1 -> Transfer Fcn2/1
  Transfer Fcn/1 -> Gain10/1, Scope7/1, Gain9/1
  Transfer Fcn2/1 -> Rear Steering Angle/1
  Gain12/1 -> Derivative2/1
  V_SA/1 -> Gain14/1
  Gain13/1 -> Sum3/3
  Gain14/1 -> Scope10/1, Gain13/1, Gain12/1
  Manual Switch (AYC ON/OFF)1/1 -> Yaw Control Signal/1
  Derivative2/1 -> Sum3/4

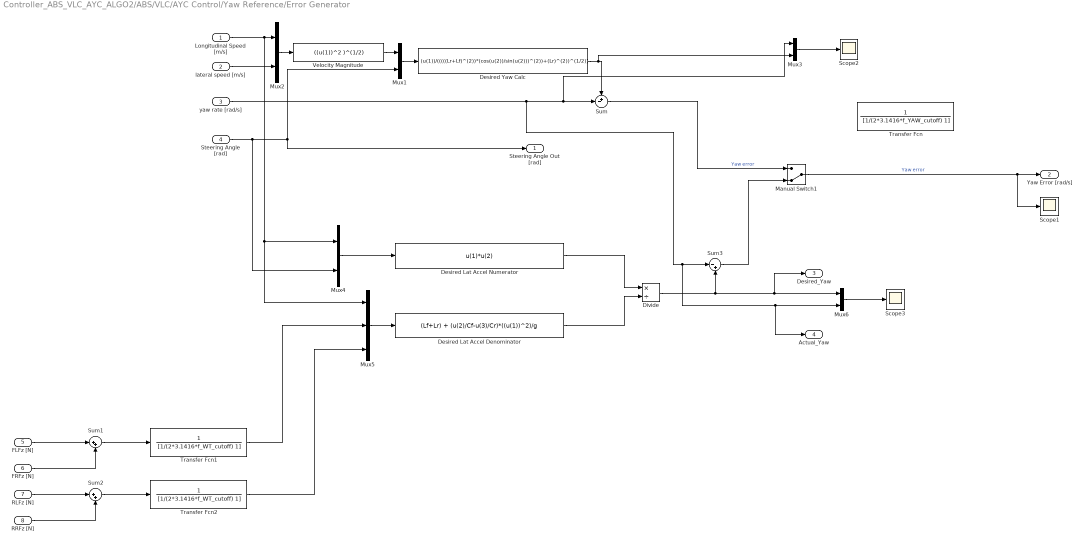
== system Controller_ABS_VLC_AYC_ALGO2/ABS/VLC/AYC Control/Yaw Reference/Error Generator ==
  Longitudinal Speed [m/s] : Inport
  lateral speed [m/s] : Inport  Port=2
  yaw rate [rad/s] : Inport  Port=3
  Steering Angle [rad] : Inport  Port=4
  FLFz [N] : Inport  Port=5
  FRFz [N] : Inport  Port=6
  RLFz [N] : Inport  Port=7
  RRFz [N] : Inport  Port=8
  Desired Lat Accel Denominator : Fcn  Expr=(Lf+Lr) + (u(2)/Cf-u(3)/Cr)*((u(1))^2)/g
  Desired Lat Accel Numerator : Fcn  Expr=u(1)*u(2)
  Desired Yaw Calc : Fcn  Expr=(u(1))/(((((Lr+Lf)^(2))*(cos(u(2))/sin(u(2)))^(2))+(Lr)^(2))^(1/2))
  Divide : Product  Inputs=*/
  Manual Switch1 : ManualSwitch  CurrentSetting=0
  Mux{1..4,6} (5 alike) : Mux  Inputs=2
  Mux5 : Mux  Inputs=3
  Scope1 : Scope
  Scope2 : Scope
  Scope3 : Scope
  Sum : Sum  Inputs=+-|
  Sum1 : Sum  Inputs=|++
  Sum2 : Sum  Inputs=|++
  Sum3 : Sum  Inputs=|-+
  Transfer Fcn : TransferFcn  Denominator=[1/(2*3.1416*f_YAW_cutoff) 1]
  Transfer Fcn1 : TransferFcn  Denominator=[1/(2*3.1416*f_WT_cutoff) 1]
  Transfer Fcn2 : TransferFcn  Denominator=[1/(2*3.1416*f_WT_cutoff) 1]
  Velocity Magnitude : Fcn  Expr=((u(1))^2 )^(1/2)
  Steering Angle Out [rad] : Outport
  Yaw Error [rad/s] : Outport  Port=2
  Desired_Yaw : Outport  Port=3
  Actual_Yaw : Outport  Port=4
  wires:
  Mux1/1 -> Desired Yaw Calc/1
  lateral speed [m/s]/1 -> Mux2/2
  Mux2/1 -> Velocity Magnitude/1
  Velocity Magnitude/1 -> Mux1/1
  Steering Angle [rad]/1 -> Mux4/2, Mux1/2, Steering Angle Out [rad]/1
  yaw rate [rad/s]/1 -> Actual_Yaw/1, Mux6/2, Sum3/1, Sum/2, Mux3/1
  Desired Yaw Calc/1 -> Sum/1, Mux3/2
  Mux3/1 -> Scope2/1
  Desired Lat Accel Numerator/1 -> Divide/1
  Desired Lat Accel Denominator/1 -> Divide/2
  Longitudinal Speed [m/s]/1 -> Mux5/1, Mux4/1, Mux2/1
  Mux4/1 -> Desired Lat Accel Numerator/1
  FLFz [N]/1 -> Sum1/1
  FRFz [N]/1 -> Sum1/2
  Sum1/1 -> Transfer Fcn1/1
  RLFz [N]/1 -> Sum2/1
  RRFz [N]/1 -> Sum2/2
  Sum2/1 -> Transfer Fcn2/1
  Mux5/1 -> Desired Lat Accel Denominator/1
  Manual Switch1/1 -> Yaw Error [rad/s]/1, Scope1/1  "Yaw error"
  Sum/1 -> Manual Switch1/1  "Yaw error"
  Divide/1 -> Desired_Yaw/1, Mux6/1, Sum3/2
  Sum3/1 -> Manual Switch1/2
  Mux6/1 -> Scope3/1
  Transfer Fcn1/1 -> Mux5/2
  Transfer Fcn2/1 -> Mux5/3
